simulink model "practice_final_part_1"  (Simulink 8.0)
settings: Solver=ode45  StartTime=0.0  StopTime=20  RelTol=1e-3
undefined symbols (not defined in the file or in its folder): drawRodMass
settings Model: Creator=beard  LastModifiedBy=tmclain
settings DataIOCC: LimitDataPoints=off  SignalLoggingSaveFormat=ModelDataLogs
settings DebuggingCC: SolverPrmCheckMsg=none  FcnCallInpInsideContextMsg=UseLocalSettings  StrictBusMsg=Warning
settings GRTTargetCC: CombineOutputUpdateFcns=off  GRTInterface=on

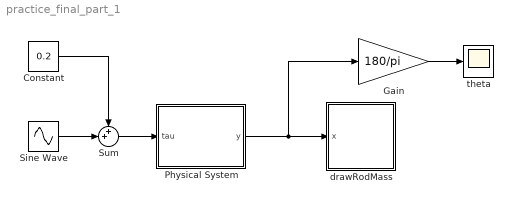
== system practice_final_part_1 ==
  Constant : Constant  Value=0.2
  Gain : Gain  Gain=180/pi
  Physical System : Subsystem
  Sine Wave : Sin  Amplitude=0.04  Frequency=pi  SampleTime=0
  Sum : Sum  Inputs=++|
  drawRodMass : Subsystem
      mask init:
      | % drawing parameters
      | L = 1;
      | w = 0.01;
      | R = 0.1;
      | H = 1;
      mask Display: image(imread('tv.jpg'))
  theta : Scope
      settings: TimeRange=20  YMin=-75  YMax=225
  wires:
  Gain/1 -> theta/1
  Physical System/1(y) -> drawRodMass/1(x), Gain/1
  Constant/1 -> Sum/1
  Sum/1 -> Physical System/1(tau)
  Sine Wave/1 -> Sum/2

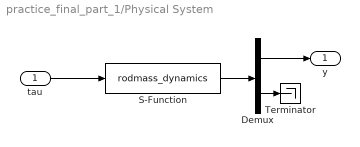
== system practice_final_part_1/Physical System ==
  tau : Inport
  Demux : Demux  Outputs=[1;2]
  S-Function : S-Function  FunctionName=rodmass_dynamics  Parameters=P  EnableBusSupport=off
  Terminator : Terminator
  y : Outport
  wires:
  tau/1 -> S-Function/1
  S-Function/1 -> Demux/1
  Demux/2 -> Terminator/1
  Demux/1 -> y/1

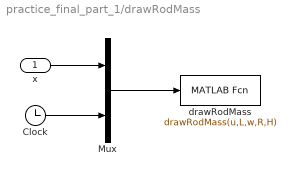
== system practice_final_part_1/drawRodMass ==
  x : Inport
  Clock : Clock
  Mux : Mux  Inputs=2
  drawRodMass : MATLABFcn  MATLABFcn=drawRodMass(u,L,w,R,H)  OutputDimensions=0  SampleTime=0.1
  wires:
  Clock/1 -> Mux/2
  x/1 -> Mux/1
  Mux/1 -> drawRodMass/1
